simulink model "testt"  (R2018a)
settings: Solver=VariableStepAuto  StartTime=0.0  StopTime=10  RelTol=1e-3
values from neighbouring files (symbols this model uses):
  b = 1    [ksi0.m]    (also in ksi05.m; ksi3.m; main.m; test.m)
  ksi = 0    [ksi0.m]    (also in ksi05.m = -1.5; ksi3.m = 1.5; main.m = 0.5; test.m = 0.1)
  w = 1.5    [ksi0.m]    (also in ksi05.m; ksi3.m; main.m; test.m = 2)
settings Model: Creator=john  LastModifiedBy=johnb

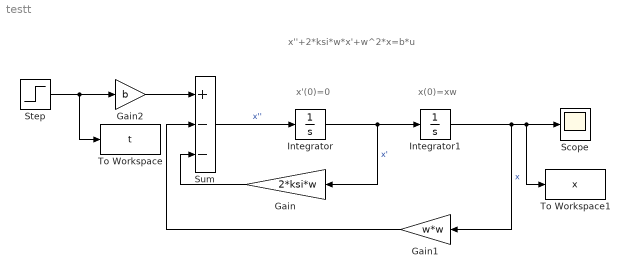
== system testt ==
  note: x(0)=xw
  note: x'(0)=0
  note: x''+2*ksi*w*x'+w^2*x=b*u
  Gain : Gain  Gain=2*ksi*w
  Gain1 : Gain  Gain=w*w
  Gain2 : Gain  Gain=b
  Integrator : Integrator
  Integrator1 : Integrator  InitialCondition=1
  Scope : Scope
  Step : Step  Before=1  SampleTime=0
  Sum : Sum  Inputs=+--
  To Workspace : ToWorkspace  VariableName=t  SaveFormat=Timeseries  SampleTime=-1
  To Workspace1 : ToWorkspace  VariableName=x  SampleTime=-1
  wires:
  Integrator/1 -> Gain/1, Integrator1/1  "x'"
  Integrator1/1 -> Gain1/1, To Workspace1/1, Scope/1  "x"
  Sum/1 -> Integrator/1  "x''"
  Gain/1 -> Sum/3
  Gain1/1 -> Sum/2
  Step/1 -> To Workspace/1, Gain2/1
  Gain2/1 -> Sum/1
